simulink model "facedetection_raspi"  (R2021b)
settings: Solver=FixedStepAuto  StartTime=0.0  StopTime=10.0  RelTol=1e-3  EnableMultiTasking=on
libraries: raspberrypiBasiclib x4, raspberrypiNetworklib x1
settings Model: Creator=86139  LastModifiedBy=86139
settings SolverCC: PositivePriorityOrder=on
settings OptimizationCC: EnhancedBackFolding=on  PassReuseOutputArgsAs=Individual arguments  ZeroExternalMemoryAtStartup=off  ZeroInternalMemoryAtStartup=off  MaxStackSize=64  OptimizeBlockOrder=speed  DifferentSizesBufferReuse=on  OptimizationCustomize=off  EfficientTunableParamExpr=on
settings DebuggingCC: ParameterTunabilityLossMsg=error
settings HardwareCC: ProdBitPerPointer=32  ProdBitPerSizeT=32  ProdBitPerPtrDiffT=32  ProdLargestAtomicInteger=Long  ProdLargestAtomicFloat=Double  ProdWordSize=32  ProdLongLongMode=on  ProdHWDeviceType=ARM Compatible->ARM Cortex  UseEmbeddedCoderFeatures=off
settings RTWCC: Description=Embedded Coder  SystemTargetFile=ert.tlc  HardwareBoard=Raspberry Pi  TLCOptions="-aInlineSetEventsForThisBaseRateFcn=TLC_FALSE -aSuppressMultiTaskScheduler=TLC_FALSE  -aRateBasedStepFcn=0"  TemplateMakefile=ert_default_tmf  Toolchain=GNU GCC Embedded Linux  BuildConfiguration=Faster Runs
settings CodeAppCC: ForceParamTrailComments=on  IgnoreCustomStorageClasses=off  OperatorAnnotations=on  SimulinkDataObjDesc=on  SFDataObjDesc=on  InsertBlockDesc=on
settings ERTTargetCC: SupportNonInlinedSFcns=on  SupportVariableSizeSignals=on  ExtModeTransport=2  ExtModeStaticAlloc=on  ExtModeMexFile=ext_xcp  ExtModeIntrfLevel=Level2 - Open

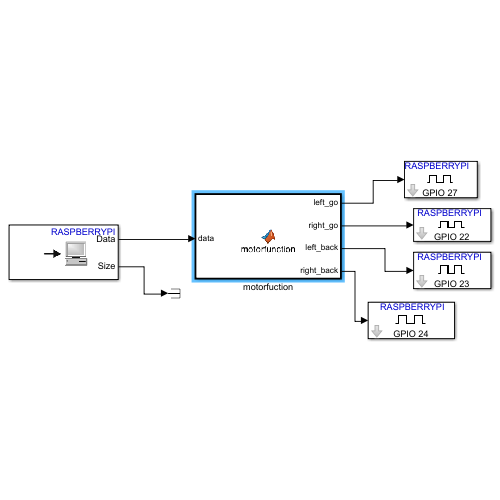
[thumbnail: Simulink's stored preview of the top-level diagram]
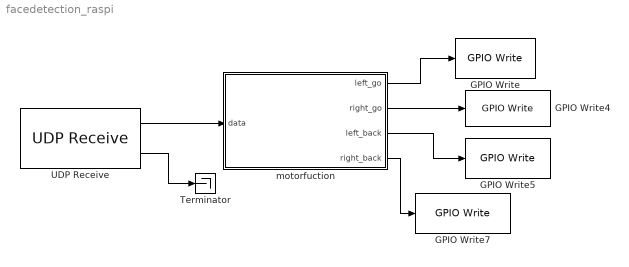
== system facedetection_raspi ==
  GPIO Write : raspberrypiBasiclib/GPIO Write  board=Pi 3 Model B  gpio=27  direction=Output  blockPlatform=Raspberry Pi
      settings: SourceProductBaseCode=RASPPI
  GPIO Write4 : raspberrypiBasiclib/GPIO Write  board=Pi 3 Model B  gpio=22  direction=Output  blockPlatform=Raspberry Pi
      settings: SourceProductBaseCode=RASPPI
  GPIO Write5 : raspberrypiBasiclib/GPIO Write  board=Pi 3 Model B  gpio=23  direction=Output  blockPlatform=Raspberry Pi
      settings: SourceProductBaseCode=RASPPI
  GPIO Write7 : raspberrypiBasiclib/GPIO Write  board=Pi 3 Model B  gpio=24  direction=Output  blockPlatform=Raspberry Pi
      settings: SourceProductBaseCode=RASPPI
  Terminator : Terminator
  UDP Receive : raspberrypiNetworklib/UDP Receive  localURL='0.0.0.0'  localPort=25000  remoteURL='0.0.0.0'  remotePort=-1  recvBufferSize=8192  signalDatatype=single  dims=255  isVarSize=off  showBlockingTime=off  blockingTime=0  sampletime=0.01  blockPlatform=Raspberry Pi
      settings: SourceProductBaseCode=RASPPI
  motorfuction : MATLAB Function  TreatAsAtomicUnit=on
  wires:
  UDP Receive/2 -> Terminator/1
  UDP Receive/1 -> motorfuction/1(data)
  motorfuction/1(left_go) -> GPIO Write/1
  motorfuction/2(right_go) -> GPIO Write4/1
  motorfuction/3(left_back) -> GPIO Write5/1
  motorfuction/4(right_back) -> GPIO Write7/1

== matlab function facedetection_raspi/motorfuction ==
  data: data input; left_go output; right_go output; left_back output; right_back output
function [left_go,right_go,left_back,right_back] = motorfunction(data)

left_go = true;
left_back = false;
right_go = true;
right_back = false;

if data == 0
    left_go = false;
    right_go = false;
    left_back = false;
    right_back = false;
end
if data == 1
    left_go = true;
    right_go = true;
    left_back = false;
    right_back = false;
end
if data == 2
    left_go = false;
    right_go = true;
    left_back = true;
    right_back = false;
end
if data == 3
    left_go = true;
    right_go = false;
    left_back = false;
    right_back = true;
end
